simulink model "ex4"  (R2020a)
settings: Solver=VariableStepAuto  StartTime=0.0  StopTime=10.0  RelTol=1e-3
libraries: simulink x2
settings Model: Creator=Kundan Patil  LastModifiedBy=Kundan Patil

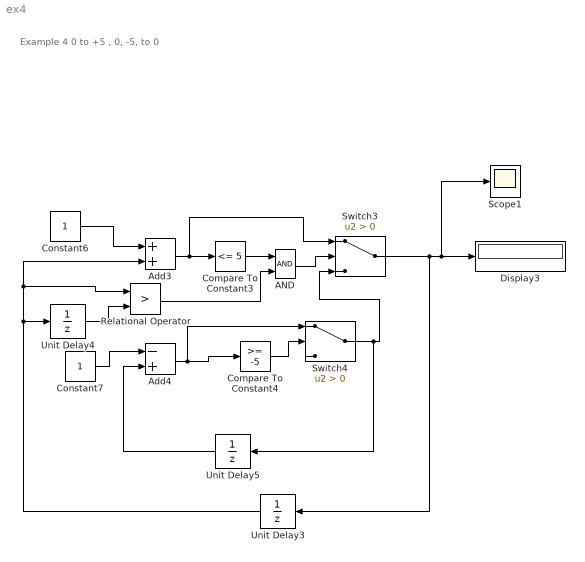
== system ex4 ==
  note: Example 4
      | 0 to +5 , 0,  -5, to 0
  AND : Logic  AllPortsSameDT=off  OutDataTypeStr=boolean
  Add3 : Sum
  Add4 : Sum  Inputs=-+
  Compare To Constant3 : simulink/Logic and Bit Operations/Compare To Constant  relop=<=  const=5  OutDataTypeStr=boolean
  Compare To Constant4 : simulink/Logic and Bit Operations/Compare To Constant  relop=>=  const=-5  OutDataTypeStr=boolean
  Constant6 : Constant
  Constant7 : Constant
  Display3 : Display
  Relational Operator : RelationalOperator  Operator=>  OutDataTypeStr=boolean  RndMeth=Simplest
  Scope1 : Scope
  Switch3 : Switch  Criteria=u2 > Threshold
  Switch4 : Switch  Criteria=u2 > Threshold
  Unit Delay3 : UnitDelay  InitialCondition=-1  SampleTime=-1  HasFrameUpgradeWarning=on
  Unit Delay4 : UnitDelay  InitialCondition=-2  SampleTime=-1  HasFrameUpgradeWarning=on
  Unit Delay5 : UnitDelay  InitialCondition=1  SampleTime=-1  HasFrameUpgradeWarning=on
  wires:
  Switch3/1 -> Unit Delay3/1, Scope1/1, Display3/1
  Constant6/1 -> Add3/1
  AND/1 -> Switch3/2
  Compare To Constant4/1 -> Switch4/2
  Switch4/1 -> Unit Delay5/1, Switch3/3
  Unit Delay5/1 -> Add4/2
  Compare To Constant3/1 -> AND/1
  Constant7/1 -> Add4/1
  Add4/1 -> Switch4/1, Compare To Constant4/1
  Add3/1 -> Switch3/1, Compare To Constant3/1
  Unit Delay4/1 -> Relational Operator/2
  Unit Delay3/1 -> Unit Delay4/1, Relational Operator/1, Add3/2
  Relational Operator/1 -> AND/2
